simulink model "AFSMC_R2020a"  (R2020b)
settings: Solver=ode4  StartTime=0.0  StopTime=100  FixedStep=0.005  RelTol=1e-3
settings Model: Creator=Dell Precision  LastModifiedBy=Dell Precision

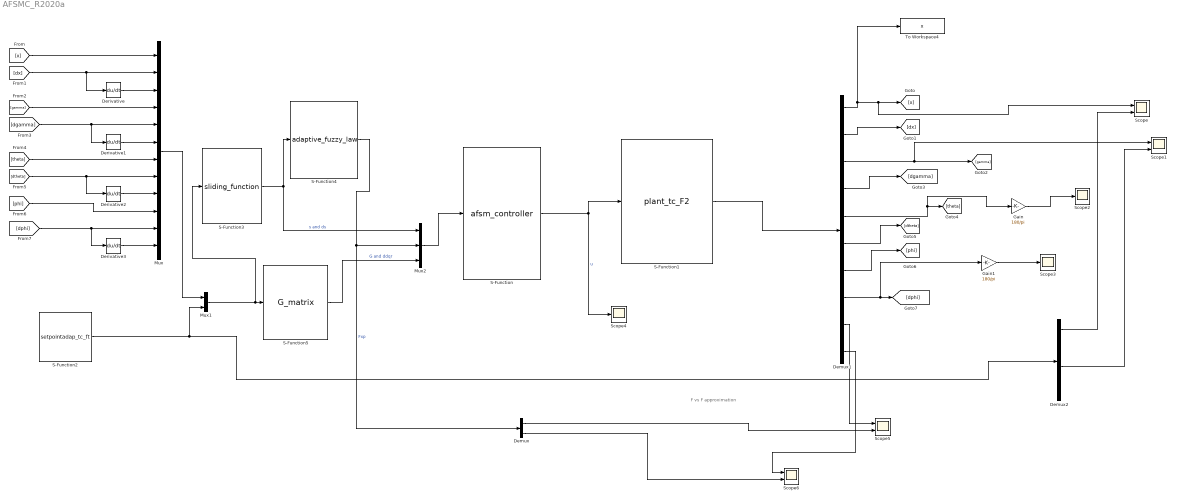
== system AFSMC_R2020a ==
  note: F vs F approximation
  Demux : Demux  Outputs=2
  Demux1 : Demux  Outputs=10
  Demux2 : Demux  Outputs=6
  Derivative{,1..3} (4 alike) : Derivative
  Gain : Gain  Gain=180/pi
  Gain1 : Gain  Gain=180/pi
  Mux : Mux  Inputs=12
  Mux1 : Mux  Inputs=2
  Mux2 : Mux  Inputs=3
  S-Function : S-Function  FunctionName=afsm_controller  SFunctionDeploymentMode=off  EnableBusSupport=off
  S-Function1 : S-Function  FunctionName=plant_tc_F2  SFunctionDeploymentMode=off  EnableBusSupport=off
  S-Function2 : S-Function  FunctionName=setpointadap_tc_ft  SFunctionDeploymentMode=off  EnableBusSupport=off
  S-Function3 : S-Function  FunctionName=sliding_function  SFunctionDeploymentMode=off  EnableBusSupport=off
  S-Function4 : S-Function  FunctionName=adaptive_fuzzy_law  SFunctionDeploymentMode=off  EnableBusSupport=off
  S-Function5 : S-Function  FunctionName=G_matrix  SFunctionDeploymentMode=off  EnableBusSupport=off
  Scope{,1,5..6} (4 alike) : Scope  NumInputPorts=2
  Scope2 : Scope
  Scope3 : Scope
  Scope4 : Scope
  To Workspace4 : ToWorkspace  VariableName=x  SaveFormat=Timeseries  SampleTime=-1
  wires:
  Demux1/9 -> Scope5/1
  Demux1/5 -> Gain/1, [theta]
  [theta] -> Mux/7
  Demux1/2 -> [dx]
  Demux1/4 -> [dgamma]
  [dphi] -> Mux/11, Derivative3/1
  [phi] -> Mux/10
  Demux1/7 -> [phi]
  Demux1/3 -> Scope1/1, [gamma]
  Demux1/8 -> Gain1/1, [dphi]
  Gain1/1 -> Scope3/1
  Demux1/10 -> Scope6/1
  Derivative/1 -> Mux/3
  [x] -> Mux/1
  Derivative2/1 -> Mux/9
  Demux2/1 -> Scope/2
  S-Function2/1 -> Demux2/1, Mux1/2
  Gain/1 -> Scope2/1
  Demux1/6 -> [dtheta]
  Derivative1/1 -> Mux/6
  [gamma] -> Mux/4
  [dgamma] -> Derivative1/1, Mux/5
  Mux/1 -> Mux1/1
  Demux1/1 -> To Workspace4/1, Scope/1, [x]
  [dx] -> Derivative/1, Mux/2
  [dtheta] -> Mux/8, Derivative2/1
  Derivative3/1 -> Mux/12
  Demux2/4 -> Scope1/2
  S-Function1/1 -> Demux1/1
  S-Function/1 -> S-Function1/1, Scope4/1  "u"
  Mux1/1 -> S-Function3/1, S-Function5/1
  S-Function3/1 -> Mux2/1, S-Function4/1  "s and ds"
  S-Function4/1 -> Mux2/2, Demux/1  "Fxp"
  S-Function5/1 -> Mux2/3  "G and ddqr"
  Mux2/1 -> S-Function/1
  Demux/1 -> Scope5/2
  Demux/2 -> Scope6/2
